simulink subsystem "Wipers_InputAquisition"  (R2025b)
settings: Solver=VariableStepAuto  StartTime=0.0  StopTime=10.0  RelTol=1e-3
libraries: simulink x7
settings Model: Creator=Sai Krishna  LastModifiedBy=Sai Krishna

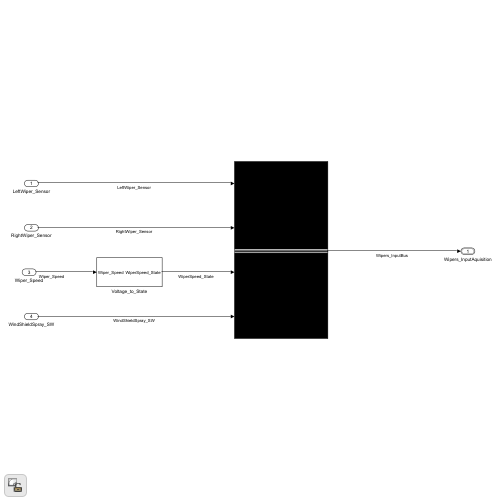
[thumbnail: Simulink's stored preview of the top-level diagram]
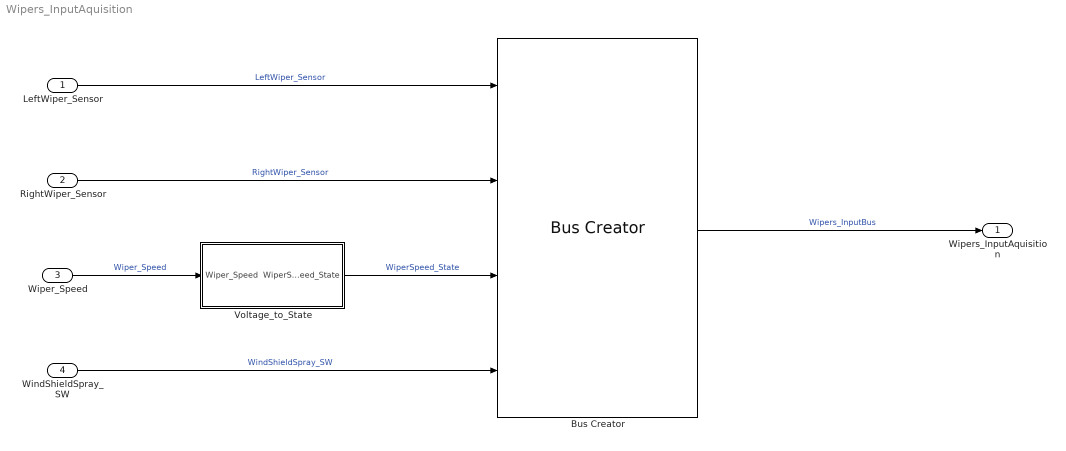
== system Wipers_InputAquisition ==
  LeftWiper_Sensor : Inport  OutDataTypeStr=boolean
  RightWiper_Sensor : Inport  Port=2  OutDataTypeStr=boolean
  Wiper_Speed : Inport  Port=3  OutDataTypeStr=double
  WindShieldSpray_SW : Inport  Port=4  OutDataTypeStr=boolean
  Bus Creator : BusCreator  Inputs=4  OutDataTypeStr=Bus: Wipers_InputBus
  Voltage_to_State : Subsystem
  Wipers_InputAquisition : Outport  OutDataTypeStr=Bus: Wipers_InputBus
  wires:
  LeftWiper_Sensor/1 -> Bus Creator/1  "LeftWiper_Sensor"
  RightWiper_Sensor/1 -> Bus Creator/2  "RightWiper_Sensor"
  WindShieldSpray_SW/1 -> Bus Creator/4  "WindShieldSpray_SW"
  Wiper_Speed/1 -> Voltage_to_State/1(Wiper_Speed)  "Wiper_Speed"
  Voltage_to_State/1(WiperSpeed_State) -> Bus Creator/3  "WiperSpeed_State"
  Bus Creator/1 -> Wipers_InputAquisition/1  "Wipers_InputBus"

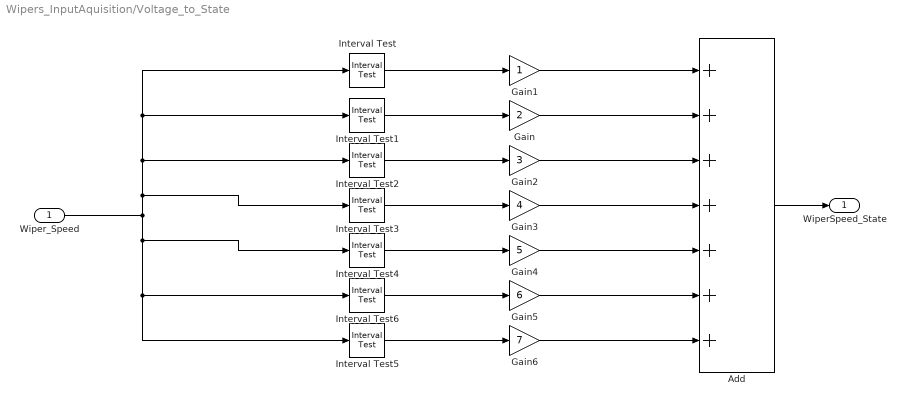
== system Wipers_InputAquisition/Voltage_to_State ==
  Wiper_Speed : Inport  OutDataTypeStr=double
  Add : Sum  Inputs=+++++++
  Gain : Gain  Gain=2  OutDataTypeStr=uint8
  Gain1 : Gain  OutDataTypeStr=uint8
  Gain2 : Gain  Gain=3  OutDataTypeStr=uint8
  Gain3 : Gain  Gain=4  OutDataTypeStr=uint8
  Gain4 : Gain  Gain=5  OutDataTypeStr=uint8
  Gain5 : Gain  Gain=6  OutDataTypeStr=uint8
  Gain6 : Gain  Gain=7  OutDataTypeStr=uint8
  Interval Test : simulink/Logic and Bit Operations/Interval Test  IntervalClosedRight=on  uplimit=1  IntervalClosedLeft=on  lowlimit=0.2  OutDataTypeStr=boolean
  Interval Test1 : simulink/Logic and Bit Operations/Interval Test  IntervalClosedRight=on  uplimit=2  IntervalClosedLeft=on  lowlimit=1.2  OutDataTypeStr=boolean
  Interval Test2 : simulink/Logic and Bit Operations/Interval Test  IntervalClosedRight=on  uplimit=3  IntervalClosedLeft=on  lowlimit=2.2  OutDataTypeStr=boolean
  Interval Test3 : simulink/Logic and Bit Operations/Interval Test  IntervalClosedRight=on  uplimit=4  IntervalClosedLeft=on  lowlimit=3.2  OutDataTypeStr=boolean
  Interval Test4 : simulink/Logic and Bit Operations/Interval Test  IntervalClosedRight=on  uplimit=5  IntervalClosedLeft=on  lowlimit=4.2  OutDataTypeStr=boolean
  Interval Test5 : simulink/Logic and Bit Operations/Interval Test  IntervalClosedRight=on  uplimit=7  IntervalClosedLeft=on  lowlimit=6.2  OutDataTypeStr=boolean
  Interval Test6 : simulink/Logic and Bit Operations/Interval Test  IntervalClosedRight=on  uplimit=6  IntervalClosedLeft=on  lowlimit=5.2  OutDataTypeStr=boolean
  WiperSpeed_State : Outport
  wires:
  Add/1 -> WiperSpeed_State/1
  Wiper_Speed/1 -> Interval Test4/1, Interval Test6/1, Interval Test5/1, Interval Test3/1, Interval Test2/1, Interval Test1/1, Interval Test/1
  Interval Test5/1 -> Gain6/1
  Interval Test6/1 -> Gain5/1
  Interval Test4/1 -> Gain4/1
  Interval Test3/1 -> Gain3/1
  Interval Test2/1 -> Gain2/1
  Interval Test1/1 -> Gain/1
  Gain6/1 -> Add/7
  Gain5/1 -> Add/6
  Gain4/1 -> Add/5
  Gain3/1 -> Add/4
  Gain2/1 -> Add/3
  Gain/1 -> Add/2
  Gain1/1 -> Add/1
  Interval Test/1 -> Gain1/1
